simulink model "balance_beam"  (R2012b)
settings: Solver=ode3  StartTime=0.0  StopTime=inf  FixedStep=0.001  RelTol=1e-3
undefined symbols (not defined in the file or in its folder): HIL
libraries: quarc_library x5
settings Model: SimulationMode=external  ExtModeTrigDuration=5000  Creator=prakrit.shrestha  LastModifiedBy=prakrit.shrestha
settings SolverCC: PositivePriorityOrder=on
settings RTWCC: SystemTargetFile=quarc_win64.tlc  TemplateMakefile=quarc_default_tmf  Description=QUARC Win64 Target  ProcessScript=quarc_win64_make_rtw_hook
settings STFCustomTargetCC: TargetPreCompLibLocation=C:\PROGRA~3\QUARC\lib\2012b\win64\release  CodeReplacementLibrary=ANSI_C  GeneratePreprocessorConditionals=Disable all  CombineOutputUpdateFcns=on  GRTInterface=off  SystemTargetFile=quarc_win64.tlc
settings GRTTargetCC: TargetPreCompLibLocation=C:\PROGRA~3\QUARC\lib\2012b\win64\release  ParMdlRefBuildCompliant=off  CompOptLevelCompliant=off  ConcurrentExecutionCompliant=off  MatFileLogging=off  ExtMode=on  ExtModeMexFile=quarc_comm

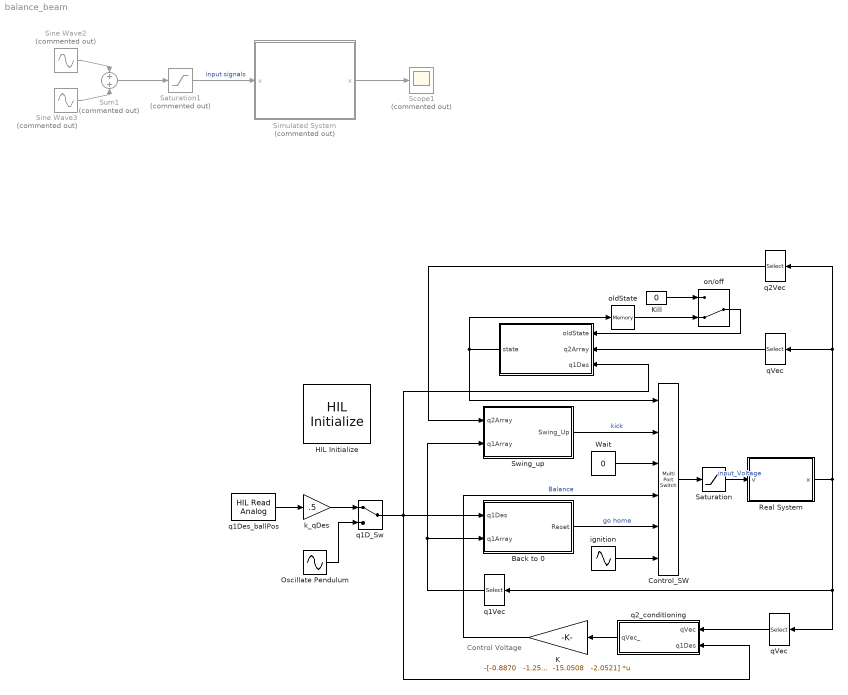
== system balance_beam ==
  note: Control Voltage
  " " : MATLAB Function  TreatAsAtomicUnit=on
  "Back to 0 " : Subsystem
  Control_SW : MultiPortSwitch  Inputs=5
  HIL Initialize : quarc_library/Data Acquisition/Generic/Configuration/HIL Initialize  Priority=-99  object_name=HIL-1  board_type=q2_usb  board_number=0  board_options=d0=digital;d1=digital;led=auto;update_rate=normal;decimation=1  exclusive=off  active=off  hardware_clocks=[0]  clock_modes=[]  initial_clock_frequencies=[]  set_clock_params_at_start=off  set_clock_params_at_switch_in=off  set_clock_frequencies_at_start=off  set_clock_frequencies_at_switch_in=off  analog_input_channels=[0:1]  analog_input_maximums=10  analog_input_minimums=-10  set_analog_input_params_at_start=on  set_analog_input_params_at_switch_in=off  analog_output_channels=[0:1]  analog_output_maximums=10  analog_output_minimums=-10  initial_analog_outputs=[0]  final_analog_outputs=[0]  watchdog_analog_outputs=0  set_analog_output_params_at_start=on  set_analog_output_params_at_switch_in=off  set_analog_outputs_at_start=on  set_analog_outputs_at_switch_in=off  set_analog_outputs_at_terminate=on  set_analog_outputs_at_switch_out=off  set_analog_outputs_on_watchdog=off  digital_input_channels=[]  digital_output_channels=[]  digital_output_configuration=[]  initial_digital_outputs=[1]  final_digital_outputs=[1]  watchdog_digital_outputs=[1]  set_digital_output_params_at_start=off  set_digital_output_params_at_switch_in=off  set_digital_outputs_at_start=on  set_digital_outputs_at_switch_in=off  set_digital_outputs_at_terminate=on  set_digital_outputs_at_switch_out=off  set_digital_outputs_on_watchdog=off  encoder_channels=[0:1]  quadrature=[4]  encoder_filter_frequency=[]  initial_encoder_counts=[0]  set_encoder_params_at_start=on  set_encoder_params_at_switch_in=off  set_encoder_counts_at_start=on  set_encoder_counts_at_switch_in=off  pwm_channels=[]  pwm_modes=[0]  pwm_frequency=1/0.020  pwm_configuration=[]  pwm_alignment=[]  pwm_polarity=[]  pwm_leading_deadband=[]  pwm_trailing_deadband=[]  initial_pwm_outputs=[0]  final_pwm_outputs=[0]  watchdog_pwm_outputs=[0]  set_pwm_params_at_start=on  set_pwm_params_at_switch_in=off  set_pwm_outputs_at_start=on  set_pwm_outputs_at_switch_in=off  set_pwm_outputs_at_terminate=on  set_pwm_outputs_at_switch_out=off  set_pwm_outputs_on_watchdog=off  other_output_channels=[]  initial_other_outputs=[]  final_other_outputs=[]  watchdog_other_outputs=[]  set_other_outputs_at_start=off  set_other_outputs_at_switch_in=off  set_other_outputs_at_terminate=off  set_other_outputs_at_switch_out=off  set_other_outputs_on_watchdog=off
  K : Gain  Gain="-[-0.8870   -1.2505  -15.0508   -2.0521]"  Multiplication=Matrix(K*u)
  "Kill " : Constant  Value=0
  Oscillate Pendulum : Sin  Frequency=10  SampleTime=0
  Real System : Subsystem
  Saturation : Saturate  UpperLimit=10  LowerLimit=-10
  Saturation1 : Saturate  Commented=on  UpperLimit=10  LowerLimit=-10
  Scope1 : Scope  Commented=on
      settings: ShowLegends=on  YMin=-60  YMax=70  SaveName=data1  MaxDataPoints=10001
  Simulated System : Subsystem  Commented=on
  Sine Wave2 : Sin  Commented=on  Amplitude=5  Frequency=13  SampleTime=0
  Sine Wave3 : Sin  Commented=on  Amplitude=8  Frequency=7  Phase=pi/4  SampleTime=0
  Sum1 : Sum  Commented=on
  "Swing_up " : Subsystem
  Wait : Constant  Value=0
  ignition : Sin  Amplitude=7  Frequency=13  SampleTime=0
  "k_qDes " : Gain  Gain=.5
  oldState : Memory  X0=5
  "on/off " : ManualSwitch  CurrentSetting=0
  q1D_Sw : ManualSwitch
  q1Des_ballPos : quarc_library/Data Acquisition/Generic/Immediate I//O/HIL Read Analog  object_name=HIL-1  channels=0  sample_time=qc_get_step_size  active=on  vector_output=off
  q1Vec : Selector  InputPortWidth=5  IndexOptions=Index vector (dialog)  Indices=[2,3]  OutputSizes=1
  q2Vec : Selector  InputPortWidth=5  IndexOptions=Index vector (dialog)  Indices=[4,5]  OutputSizes=1
  q2_conditioning : MATLAB Function  TreatAsAtomicUnit=on
  qVec : Selector  InputPortWidth=5  IndexOptions=Index vector (dialog)  Indices=[2, 3, 4,5]  OutputSizes=1
  "qVec  " : Selector  InputPortWidth=5  IndexOptions=Index vector (dialog)  Indices=[2, 3, 4,5]  OutputSizes=1
  wires:
  Saturation/1 -> Real System/1(v)  "input_Voltage"
  Sine Wave3/1 -> Sum1/2
  Sine Wave2/1 -> Sum1/1
  Sum1/1 -> Saturation1/1
  Saturation1/1 -> Simulated System/1(v)  "input signals"
  Simulated System/1(x) -> Scope1/1
  Control_SW/1 -> Saturation/1
  Wait/1 -> Control_SW/3
  " "/1(state) -> Control_SW/1, oldState/1
  q2Vec/1 -> "Swing_up "/1(q2Array)
  q1Vec/1 -> "Swing_up "/2("q1Array "), "Back to 0 "/2("q1Array ")
  "Swing_up "/1("Swing_Up ") -> Control_SW/2  "kick"
  K/1 -> Control_SW/4  "Balance"
  "qVec  "/1 -> q2_conditioning/1(qVec)
  Real System/1(x) -> q2Vec/1, qVec/1, "qVec  "/1, q1Vec/1
  q1Des_ballPos/1 -> "k_qDes "/1
  q2_conditioning/1(qVec_) -> K/1
  qVec/1 -> " "/2(q2Array)
  q1D_Sw/1 -> " "/3(q1Des), q2_conditioning/2(q1Des), "Back to 0 "/1("q1Des ")
  "Back to 0 "/1("Reset ") -> Control_SW/5  "go home"
  "k_qDes "/1 -> q1D_Sw/1
  Oscillate Pendulum/1 -> q1D_Sw/2
  ignition/1 -> Control_SW/6
  "on/off "/1 -> " "/1(oldState)
  oldState/1 -> "on/off "/2
  "Kill "/1 -> "on/off "/1

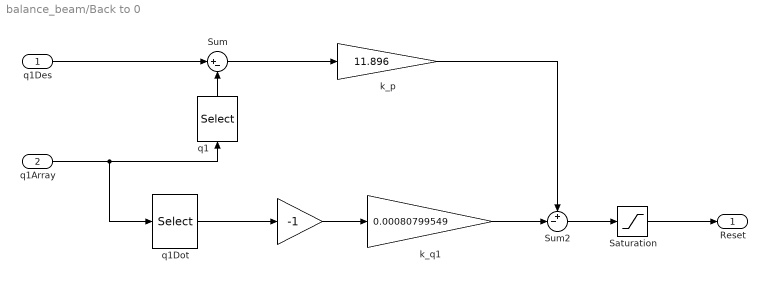
== system balance_beam/Back to 0  ==
  "q1Des " : Inport
  "q1Array " : Inport  Port=2
  "       " : Gain  Gain=-1
  Saturation : Saturate  UpperLimit=1.5  LowerLimit=-1.5
  Sum : Sum  Inputs=|+-
  Sum2 : Sum  Inputs=+-|
  k_p : Gain  Gain=11.896
  k_q1 : Gain  Gain=0.00080799549
  q1 : Selector  InputPortWidth=2  IndexOptions=Index vector (dialog)  Indices=[1]  OutputSizes=1
  q1Dot : Selector  InputPortWidth=2  IndexOptions=Index vector (dialog)  Indices=[2]  OutputSizes=1
  "Reset " : Outport
  wires:
  q1Dot/1 -> "       "/1
  "       "/1 -> k_q1/1
  Sum2/1 -> Saturation/1
  k_p/1 -> Sum2/1
  k_q1/1 -> Sum2/2
  Sum/1 -> k_p/1
  "q1Array "/1 -> q1Dot/1, q1/1
  q1/1 -> Sum/2
  Saturation/1 -> "Reset "/1
  "q1Des "/1 -> Sum/1

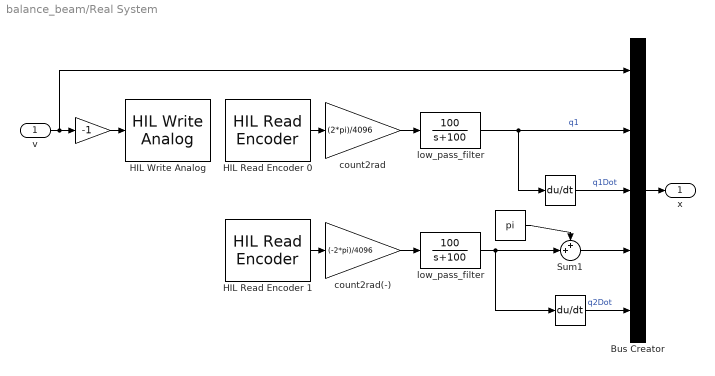
== system balance_beam/Real System ==
  v : Inport
  " " : Constant  Value=pi
  "  " : Derivative
  "   " : Derivative
  "      " : Gain  Gain=-1
  Bus Creator : BusCreator  Inputs=5
  HIL Read Encoder 0 : quarc_library/Data Acquisition/Generic/Immediate I//O/HIL Read Encoder  object_name=HIL-1  channels=0  sample_time=qc_get_step_size  active=on  vector_output=off  data_type_mode=Inherit via back propagation  data_type=double
  "HIL Read Encoder 1 " : quarc_library/Data Acquisition/Generic/Immediate I//O/HIL Read Encoder  object_name=HIL-1  channels=1  sample_time=qc_get_step_size  active=on  vector_output=off  data_type_mode=Inherit via back propagation  data_type=double
  HIL Write Analog : quarc_library/Data Acquisition/Generic/Immediate I//O/HIL Write Analog  object_name=HIL-1  channels=0  sample_time=-1  active=off  vector_input=off
  Sum1 : Sum  Inputs=++|
  "count2rad " : Gain  Gain=(2*pi)/4096
  "count2rad(-) " : Gain  Gain=(-2*pi)/4096
  low_pass_filter : TransferFcn  Numerator=[100]  Denominator=[1 100]
  "low_pass_filter " : TransferFcn  Numerator=[100]  Denominator=[1 100]
  x : Outport
  wires:
  v/1 -> "      "/1, Bus Creator/1
  "low_pass_filter "/1 -> Sum1/2, "   "/1
  " "/1 -> Sum1/1
  HIL Read Encoder 0/1 -> "count2rad "/1
  "      "/1 -> HIL Write Analog/1
  "HIL Read Encoder 1 "/1 -> "count2rad(-) "/1
  Sum1/1 -> Bus Creator/4
  "   "/1 -> Bus Creator/5  "q2Dot"
  "  "/1 -> Bus Creator/3  "q1Dot"
  Bus Creator/1 -> x/1
  "count2rad "/1 -> low_pass_filter/1
  low_pass_filter/1 -> Bus Creator/2, "  "/1  "q1"
  "count2rad(-) "/1 -> "low_pass_filter "/1

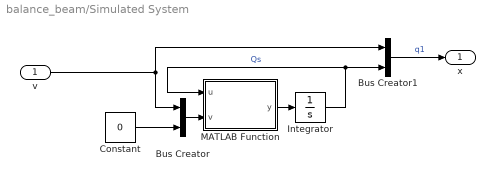
== system balance_beam/Simulated System ==
  v : Inport
  Bus Creator : BusCreator  Inputs=2
  Bus Creator1 : BusCreator  Inputs=2
  Constant : Constant  Value=0
  Integrator : Integrator  InitialCondition=[0;0;-.1;0]
  MATLAB Function : MATLAB Function  TreatAsAtomicUnit=on
  x : Outport
  wires:
  v/1 -> Bus Creator/1, Bus Creator1/1
  Bus Creator/1 -> MATLAB Function/2(v)
  Bus Creator1/1 -> x/1  "q1"
  Constant/1 -> Bus Creator/2
  Integrator/1 -> Bus Creator1/2, MATLAB Function/1(u)  "Qs"
  MATLAB Function/1(y) -> Integrator/1

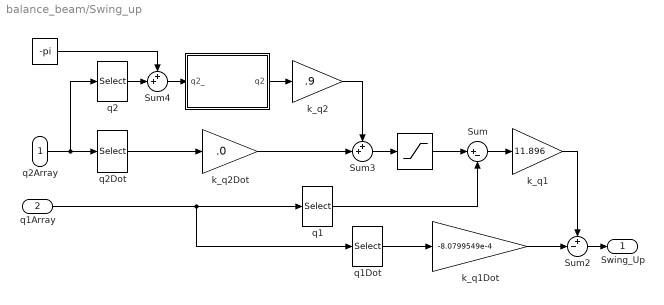
== system balance_beam/Swing_up  ==
  q2Array : Inport
  "q1Array " : Inport  Port=2
  " " : Saturate  UpperLimit=pi/6  LowerLimit=-pi/6
  "  " : MATLAB Function  TreatAsAtomicUnit=on
  "   " : Constant  Value=-pi
  Sum : Sum  Inputs=|+-
  Sum2 : Sum  Inputs=+-|
  Sum3 : Sum  Inputs=++|
  Sum4 : Sum  Inputs=++|
  "k_q1 " : Gain  Gain=11.896
  k_q1Dot : Gain  Gain=-8.0799549e-4
  k_q2 : Gain  Gain=.9
  "k_q2Dot " : Gain  Gain=.0
  "q1 " : Selector  InputPortWidth=2  IndexOptions=Index vector (dialog)  Indices=[1]  OutputSizes=1
  q1Dot : Selector  InputPortWidth=2  IndexOptions=Index vector (dialog)  Indices=[2]  OutputSizes=1
  "q2 " : Selector  InputPortWidth=2  IndexOptions=Index vector (dialog)  Indices=[1]  OutputSizes=1
  q2Dot : Selector  InputPortWidth=2  IndexOptions=Index vector (dialog)  Indices=[2]  OutputSizes=1
  "Swing_Up " : Outport
  wires:
  k_q2/1 -> Sum3/1
  "k_q2Dot "/1 -> Sum3/2
  Sum3/1 -> " "/1
  q2Dot/1 -> "k_q2Dot "/1
  "q2 "/1 -> Sum4/2
  " "/1 -> Sum/1
  Sum4/1 -> "  "/1(q2_)
  "   "/1 -> Sum4/1
  "q1Array "/1 -> "q1 "/1, q1Dot/1
  "  "/1(q2) -> k_q2/1
  Sum2/1 -> "Swing_Up "/1
  q2Array/1 -> q2Dot/1, "q2 "/1
  "k_q1 "/1 -> Sum2/1
  k_q1Dot/1 -> Sum2/2
  Sum/1 -> "k_q1 "/1
  "q1 "/1 -> Sum/2
  q1Dot/1 -> k_q1Dot/1

== matlab function balance_beam/  ==
  data: oldState input; q2Array input; state output; q1Des input
function state  = stateIdentifier(oldState, q2Array,q1Des)

state = oldState;

q1 = (q2Array(1) * 180)/ pi;    %   q1 Conditioning
q1 = abs(mod(q1, 360));

q1Desired = q1Des * 180/ pi;    %   q1Desired Conditioning

q2 = (q2Array(3) * 180)/ pi;    %   q2 Conditioning
q2 = mod(q2, 360);
q2Dot = abs(q2Array(4));

if q2 > 180
    q2 = 360 - q2;
end

if oldState == 0        %   Kill 
    state = 2;      
elseif oldState == 1    %   Swing Up
    if q2 < 30              %   if caught in state 3 domain
        state = 3;          %   go to Balance state
    end
elseif oldState == 2    %   Wait
    if (q2 > 170) && (q2Dot < 1)
        state = 4;      %	go home
    end
elseif oldState == 3    %   Balance
    if q2 > 35              %   if beam falls
        state = 2;          %   wait
    end
elseif oldState == 4    %   Homing State
    if (abs(q1-q1Desired) < 20) && (q2Dot < 0.1)    %   home yet?
        state = 1;      %   give it a kick
    end
elseif oldState == 5    %   initial kick (too lazy to move!!)
    if q2Dot > 0.5
        state = 1;
    end
end

== matlab function balance_beam/Simulated System/MATLAB Function ==
  data: u input; y output; v input
function y  =  fcn(u,v)

theta1 = 0.030372023809524;
theta2 = 0.018426339285714;
theta3 = 0.018426339285714;
theta4 = 0.092131696428571;
theta5 = 0.610144642857143;
theta6 = 0.009672619047619;

g = 9.81;

q1  =  u(1);  q1Dot  =  u(2);
q2  =  u(3);  q2Dot  =  u(4);

%u(3) is calling the third element in u matrix i.e. q2
M  = [theta1 + theta2 .* sin(q2).^2,  theta3 .* cos(q2); ...
      theta3 .* cos(q2),               theta2];

C = [2 .* theta2 .* sin(q2) .* cos(q2) * q2Dot,...
     - theta3 .* sin(q2) .* q2Dot;...
     - theta2 .* sin(q2) .* cos(q2) * q1Dot,...
    0];

F = [theta5 .* q1Dot;...
    theta6 .* q2Dot];
G = [0; ...
    - theta4 .* g .* sin(q2)];

qDot_ = [q1Dot;...
        q2Dot];
Minv = inv(M);

qDDot_ =  - Minv * (C * qDot_ + F + G) + Minv * v;

y  =  [qDot_(1);...
      qDDot_(1);...
      qDot_(2);...
      qDDot_(2)];

== matlab function balance_beam/Swing_up /   ==
  data: q2_ input; q2 output
function q2 = q2_bounded(q2_)

q2_ = mod(q2_, 2*pi); %   welcome back mod

if q2_ > pi
    q2_ = q2_ - (2*pi); %   
end

q2 = q2_;
end

== matlab function balance_beam/q2_conditioning ==
  data: qVec input; qVec_ output; q1Des input
function qVec_ = q2_real(qVec, q1Des)

    q2 = atan2(sin(qVec(3)),cos(qVec(3)));    %   polar conditioning
    q1 = qVec(1) - q1Des;

    qVec_ = [q1; qVec(2); q2; qVec(4)];
end
